simulink model "ODE_first"  (R2015a)
settings: Solver=ode4  StartTime=0.0  StopTime=3.5  RelTol=1e-3
settings Model: Creator=Kunal  LastModifiedBy=Kunal

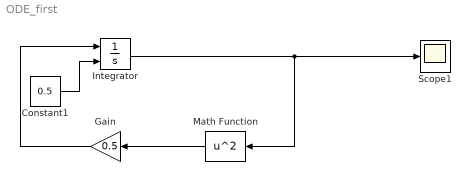
== system ODE_first ==
  Constant1 : Constant  Value=0.5
  Gain : Gain  Gain=0.5
  Integrator : Integrator  InitialConditionSource=external
  Math Function : Math  Operator=square  SaturateOnIntegerOverflow=on
  Scope1 : Scope
  wires:
  Integrator/1 -> Math Function/1, Scope1/1
  Math Function/1 -> Gain/1
  Gain/1 -> Integrator/1
  Constant1/1 -> Integrator/2
